simulink model "WashingMachine"  (R2023b)
settings: Solver=VariableStepAuto  StartTime=0.0  StopTime=inf  FixedStep=0.02  RelTol=1e-3
libraries: slpidlib x1
(part 2 of 2)

== stateflow chart WashingMachine/DES ==
  settings: enableNonTerminalStates=1
  state S3
    en:Motor_Voltage = 0;
    Swich_LR = 0;
  state STOP
  state Start
    en:Hot_Valve = 1;
    Washing = 1;
    Swich_LR = 0;
    Motor_Voltage = 0;
    Evacuation_Valve = 0;
  state S1
    en:Hot_Valve = 0;
    Cold_Valve = 1;
  state S2
    en:Cold_Valve = 0;
    Swich_LR = 1;
    Motor_Voltage = w_v;
  state S4
    en:Swich_LR = 2;
    en:Motor_Voltage = w_v;
  state S5
    en:
    Washing = 0;
    en:Swich_LR = 0;
    Motor_Voltage= 0;
  state S9
    en:Evacuation_Valve = 0;
    Swich_LR = 1;
    Motor_Voltage= s_v;
    Spin = 1;
  state S12
    en:Motor_Voltage= 0;
    Spin = 0;
    en:Swich_LR = 0;
  state S11
    en:Swich_LR = 2;
    Motor_Voltage= s_v;
  state S8
    en:Cold_Valve = 0;
    Evacuation_Valve = 1;
    Rinse = 0;
  state S6
    en:Hot_Valve = 1;
    Rinse = 1;
  state S7
    en:Hot_Valve = 0;
    Cold_Valve = 1;
  state S10
    en:Motor_Voltage = 0;
    Swich_LR = 0;
  (default) -> Start [order 1] : [start==1]
  (default) -> STOP [order 2]
  S2 -> S3 : after((w_t)/2,msec)
  S3 -> S4 : after(75,msec)
  Start -> S1 : after(h_t,msec)
  S1 -> S2 : after(c_t,msec)
  S4 -> S5 : after((w_t)/2,msec)
  S5 -> S6 : after(125,msec)
  S12 -> (junction 204)
  S11 -> S12 : after((s_t)/2,msec)
  S8 -> S9 : after(e_t,msec)
  S7 -> S8 : after(c_t,msec)
  S6 -> S7 : after(h_t,msec)
  S10 -> S11 : after(75,msec)
  S9 -> S10 : after((s_t)/2,msec)
  data: c_t input; h_t input; e_t input; s_t input; Hot_Valve output; Swich_LR output; Cold_Valve output; Washing output; Evacuation_Valve output; Rinse output double; Spin output; w_t input; start input; Motor_Voltage output; s_v input; w_v input

== matlab function WashingMachine/Processor ==
  data: w_t output; Weight input; Dirt input; RPM input; c_t output; h_t output; e_t output; s_t output; s_v output; w_v output
function [w_t,c_t,h_t,e_t,s_t,s_v,w_v] = fcn( Weight, Dirt, RPM)

 
    j=0.6;
    W = Weight*0.125;
    Wash_time = Dirt*1000;
    Hot_Water = Dirt*W;
    Cold_Water = (4-Dirt)*W;  
    Evacuation_time =  Weight*0.25;
    Spin_time = W*5;
    Spin_V = ((2*pi*RPM)/60)*1.25;
    Washing_V = Spin_V*j;


c_t = Cold_Water;
h_t = Hot_Water;
e_t = Evacuation_time;
s_t = Spin_time;
s_v = Spin_V;
w_v = Washing_V;
w_t = Wash_time;

%Hamid Reza Heidari - Control Of Mechatronic System - AmirKabir University Of Technology - 2023-16-12%
